simulink model "A9"  (R2017a)
settings: Solver=VariableStepAuto  StartTime=0.0  StopTime=0.25  MaxStep=1e-4  RelTol=1e-3
libraries: powerlib x8
settings Model: Creator=Amir Reza  LastModifiedBy=Amir Reza

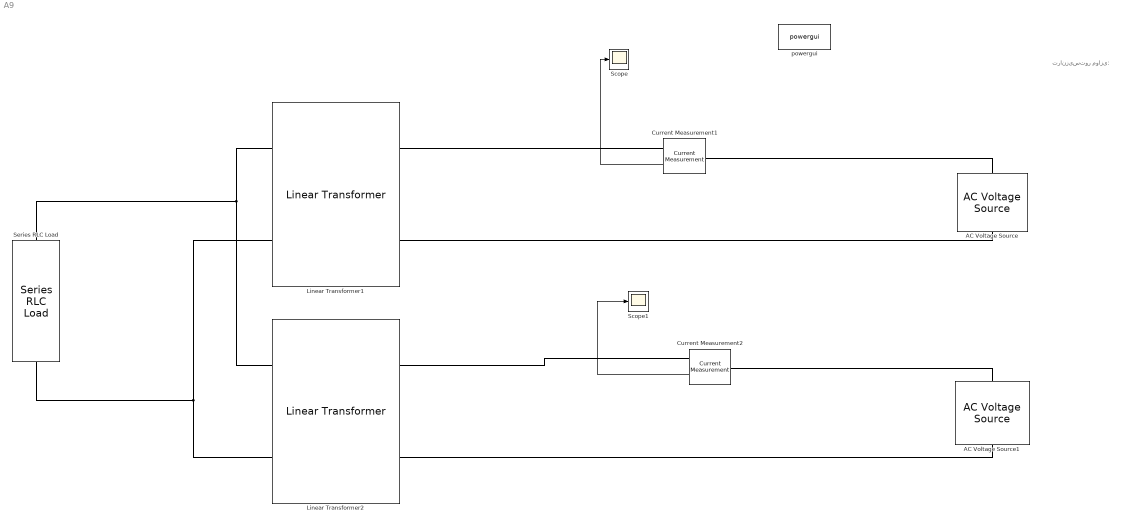
== system A9 ==
  note: ترانزیستور موازی:
  AC Voltage Source : powerlib/Electrical Sources/AC Voltage Source  Amplitude=2400  Phase=0  Frequency=50  SampleTime=0  Measurements=None  BusType=swing  Pref=10e3  Qref=0  Qmin=-inf  Qmax=+inf
  AC Voltage Source1 : powerlib/Electrical Sources/AC Voltage Source  Amplitude=2375  Phase=0  Frequency=50  SampleTime=0  Measurements=None  BusType=swing  Pref=10e3  Qref=0  Qmin=-inf  Qmax=+inf
  Current Measurement1 : powerlib/Measurements/Current Measurement  PhasorSimulation=off  OutputType=Complex  PSBequivalent=0
  Current Measurement2 : powerlib/Measurements/Current Measurement  PhasorSimulation=off  OutputType=Complex  PSBequivalent=0
  Linear Transformer1 : powerlib/Elements/Linear Transformer  UNITS=SI  NominalPower=[75e3 50 ]  winding1=[240 6e-3 7.57e-5]  winding2=[2400 0.23 9.74e-3]  ThreeWindings=off  winding3=[3.15e+05 1.0502e+06 354.69]  RmLm=[25 3.97e-2]  Measurements=None  DataType=on
  Linear Transformer2 : powerlib/Elements/Linear Transformer  UNITS=SI  NominalPower=[50e3 50 ]  winding1=[240 5.03e-3 1.098e-4]  winding2=[2375 0.384 0.011]  ThreeWindings=off  winding3=[3.15e+05 1.0502e+06 354.69]  RmLm=[25.52 4.06e-2]  Measurements=None  DataType=on
  Scope : Scope
  Scope1 : Scope
  Series RLC Load : powerlib/Elements/Series RLC Load  LConnTagsString=a  RConnTagsString=__new0  NominalVoltage=100e3  NominalFrequency=50  ActivePower=50e3  InductivePower=86.80e3  CapacitivePower=0  Setx0=off  InitialVoltage=0  SetiL0=off  InitialCurrent=0  Measurements=None  LoadType=constant Z
  powergui : powerlib/powergui  Priority=1  SimulationMode=Continuous  SampleTime=50e-6  frequency=60  Iterations=50  frequencyindice=50  Pbase=100e6  ErrMax=1e-4  UnitsV=kV  UnitsW=MW  buscounter=0  FunctionMessages=off  echomessages=off  EnableUseOfTLC=off  CurrentSourceSwitches=off  DisableSnubberDevices=off  DisableRonSwitches=off  DisableVfSwitches=off  DisplayEquations=off  SolverType=Tustin/Backward Euler (TBE)  Interpol=off  ExternalGateDelay=off  methode=off  Ts=100  x0status=blocks  SPID=on  SwTol=0  HookPort=off  RestoreLinks=warning  ResistiveCurrentMeasurement=off  Frange=[0:2:500]  Ylog=off  Xlog=on  ShowGrid=off  save=off  variable=ZData  structure=0  ZoomFFT=off  StartTime=0.0  cycles=1  DisplayStyle=1  fundamental=60  FreqAxis=off  MaxFrequency=1000  frequencyindicesteady=1  RmsSteady=1  display=off
  wires:
  Current Measurement1/1 -> Scope/1
  Current Measurement2/1 -> Scope1/1
  connections:
  AC Voltage Source1/LConn1 -- Linear Transformer2/RConn2
  Linear Transformer2/LConn2 -- Series RLC Load/RConn1 -- Linear Transformer1/LConn2
  AC Voltage Source/LConn1 -- Linear Transformer1/RConn2
  Linear Transformer1/LConn1 -- Series RLC Load/LConn1 -- Linear Transformer2/LConn1
  Linear Transformer2/RConn1 -- Current Measurement2/RConn1
  Current Measurement2/LConn1 -- AC Voltage Source1/RConn1
  Linear Transformer1/RConn1 -- Current Measurement1/RConn1
  Current Measurement1/LConn1 -- AC Voltage Source/RConn1
